simulink model "Factorial"  (R2018a)
settings: Solver=VariableStepAuto  StartTime=0.0  StopTime=10.0  RelTol=1e-3  EnableMultiTasking=on
settings Model: Creator=LEGION  LastModifiedBy=user
settings OptimizationCC: LifeSpan=inf
settings DebuggingCC: SFUnexpectedBacktrackingDiag=warning  SFNoUnconditionalDefaultTransitionDiag=warning  SFExecutionAtInitializationDiag=none
settings CodeAppCC: StateflowObjectComments=on
settings GRTTargetCC: TargetLangStandard=C89/C90 (ANSI)  GeneratePreprocessorConditionals=Disable all
settings ConfigComp: CovMetricSettings=dw  CovHtmlReporting=on  CovSaveCumulativeToWorkspaceVar=on  CovSaveSingleToWorkspaceVar=on  CovExternalEMLEnable=off

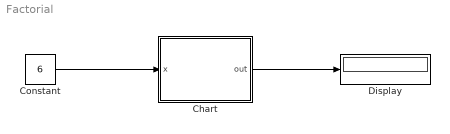
== system Factorial ==
  Chart : Stateflow chart  TreatAsAtomicUnit=on
  Constant : Constant  Value=6
  Display : Display
  wires:
  Constant/1 -> Chart/1(x)
  Chart/1(out) -> Display/1

== stateflow chart Factorial/Chart ==
  (default) -> (junction 7) : % Factorial
  (junction 7) -> (junction 9) : { n = x;,res=1;}
  (junction 9) -> (junction 8) [order 1] : [n>0]
  (junction 8) -> (junction 10) : {res = n*res;n=n-1;}
  (junction 10) -> (junction 9)
  (junction 9) -> (junction 11) [order 2] : {out = res;}
  data: x input; out output; n local; res local
